simulink model "high_level_v2"  (R2017a)
settings: Solver=FixedStepAuto  StartTime=0.0  StopTime=25  FixedStep=0.05  RelTol=1e-3
values from neighbouring files (symbols this model uses):
  Ki = 0.1419    [setup.m]
  Kia = 1.3061    [setup.m]
  kiax = 13.56    [setup.m]
  Kix = -0.08    [setup.m]
  Kpa = 1.3061    [setup.m]
  Kpax = 4.2701    [setup.m]
  Kpx = 7.1849    [setup.m]
  total_waypoints = length(xwaypoints)    [run.m]
  TxBreak = 0    [setup.m]
  TxCoulomb = 2.5    [setup.m]
  TxVisc = 49.1750    (= 49.175)    [setup.m]
  TyBreak = 0    [setup.m]
  TyCoulomb = 1.8    [setup.m]
  xwaypoints = targets(:, 1) / 100    [run.m]
  xZero = 0    [setup.m]
  ywaypoints = targets(:, 2) / 100    [run.m]
  yZero = 0.    (= 0)    [setup.m]
undefined symbols (not defined in the file or in its folder): m, MR, TzBreak, TzCoulomb, X, xRange, Y, yRange, Z, zRange, zZero
undefined symbols (not defined in the file): M, TorqueMultX, TorqueMultY, TorqueMultZ, TxTrans, TyTrans, TyVisc, TzTrans, TzVisc
libraries: sm_lib x146, fl_lib x62, nesl_utility x24, elec_lib x9, simulink x6, sm_double_wishbone_suspension_lib x4, checkpacklib x2, sharedtransform x1
(part 1 of 14)
settings Model: Creator=nadeen  LastModifiedBy=vince
settings DataIOCC: ReturnWorkspaceOutputs=on
settings ExplorerConfigSet: SimMechanicsOpenEditorOnUpdate=off

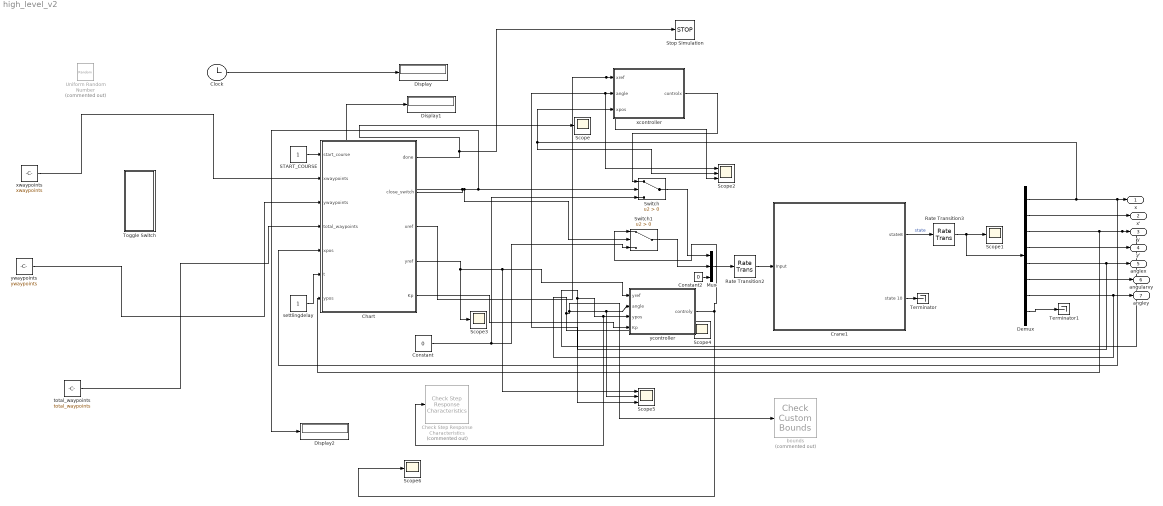
== system high_level_v2 ==
  "  bounds" : checkpacklib/Check Custom Bounds  Commented=on  InstantiateOnLoad=on  enabled=on  stopWhenAssertionFail=off  export=on  ViewDlgPos=[100.333333333333 199.666666666667 510 390]  OpenViewOnLoad=off  LaunchViewOnOpen=off  TimeUnits=seconds  EnableUpperBound=on  UpperBoundTimes=[0 2;2 7 ]  UpperBoundAmplitudes=[0.08 0.08;0.02 0.02]  EnableLowerBound=on  LowerBoundTimes=[0 2;2 7 ]  LowerBoundAmplitudes=[-0.08 -0.08;-0.02 -0.02]
  Chart : Stateflow chart  TreatAsAtomicUnit=on
  Check Step Response Characteristics : checkpacklib/Check Step Response  Characteristics  Commented=on  InstantiateOnLoad=on  enabled=on  stopWhenAssertionFail=off  export=off  ViewDlgPos=[]  OpenViewOnLoad=off  LaunchViewOnOpen=off  TimeUnits=seconds  EnableStepResponseBound=on  InitialValue=0  FinalValue=0.3  StepTime=0  RiseTime=3  PercentRise=90  SettlingTime=5  PercentSettling=0.2  PercentOvershoot=0.2  PercentUndershoot=1
  Clock : Clock
  Constant : Constant  Value=0
  Constant2 : Constant  Value=0
  Crane1 : Subsystem  mask{penduMass=m, cartMass=M, MR=MR, xRange=xRange, yRange=yRange, zRange=zRange, xZero=xZero, yZero=yZero, zZero=zZero, TxBreak=TxBreak, TxCoulomb=TxCoulomb, TxVisc=TxVisc, TxTrans=TxTrans, TyBreak=TyBreak, TyCoulomb=TyCoulomb, TyVisc=TyVisc, TyTrans=TyTrans, TzBreak=TzBreak, TzCoulomb=TzCoulomb, TzVisc=TzVisc, TzTrans=TzTrans, Ux=TorqueMultX, Uy=TorqueMultY, Uz=TorqueMultZ}
      mask prompts: penduMass "Pendulum Mass (Kg)"; cartMass "Mass of the cart (Kg)"; MR "Mass of the rail (Kg)"; TxBreak "BreakAwayFriction"; TxCoulomb "Coulomb Friction"; TxVisc "Viscous friction"; TxTrans "Transition coeff"; TyBreak "BreakAwayFriction"; TyCoulomb "Coulomb Friction"; TyVisc "Viscous friction"; TyTrans "Transition coeff"; TzBreak "BreakAwayFriction"; TzCoulomb "Coulomb Friction"; TzVisc "Viscous friction"; TzTrans "Transition coeff"; Ux "Rail motor multiplier (X)"; Uy "Cart motor multiplier (Y)"; Uz "String motor multiplier (Z)"
      mask init:
      | %mass lowSat
      | penduMass=max(penduMass,1e-3);
      | cartMass=max(cartMass,1e-3);
      | MR=max(MR,1e-3);
      | 
      | %zeros saturated
      | xZero=max(xZero,xRange(1));
      | xZero=min(xZero,xRange(2));
      | 
      | yZero=max(yZero,yRange(1));
      | yZero=min(yZero,yRange(2));
      | 
      | zZero=max(zZero,zRange(1));
      | zZero=min(zZero,zRange(2));
      mask DialogControl DescGroupVar Prompt: 3D Crane Simscape model
      mask Display:
